simulink model "statespace_verification_sim_model"  (R2016a)
settings: Solver=ode4  StartTime=0.0  StopTime=Tfinal  FixedStep=Ts  RelTol=1e-3
values from neighbouring files (symbols this model uses):
  Cdc = 15e-6    (= 1.5e-05)    [Rectifier.m]    (also in stateSpaceEnes.m; state_space_inverter.m; state_space_inverter_linetolineprinciple.m)
  DCSourceMagn = 300    [Rectifier.m]    (also in state_space_inverter.m; state_space_inverter_linetolineprinciple.m)
  delta = 0    [CapacitorAResponse.m]    (also in Rectifier.m; stateSpaceEnes.m; state_space_inverter.m; state_space_inverter_linetolineprinciple.m)
  fout = 50    [CapacitorAResponse.m]    (also in Rectifier.m; stateSpaceEnes.m; state_space_inverter.m; state_space_inverter_linetolineprinciple.m)
  GridFreq = 50    [Rectifier.m]    (also in state_space_inverter_linetolineprinciple.m)
  LA = 15e-3    (= 0.015)    [CapacitorAResponse.m]    (also in Rectifier.m; stateSpaceEnes.m; state_space_inverter.m; state_space_inverter_linetolineprinciple.m)
  LB = 15e-3    (= 0.015)    [CapacitorAResponse.m]    (also in Rectifier.m; stateSpaceEnes.m; state_space_inverter.m; state_space_inverter_linetolineprinciple.m)
  LC = 15e-3    (= 0.015)    [CapacitorAResponse.m]    (also in Rectifier.m; stateSpaceEnes.m; state_space_inverter.m; state_space_inverter_linetolineprinciple.m)
  Lin = 5e-5    (= 5e-05)    [Rectifier.m]    (also in stateSpaceEnes.m; state_space_inverter.m = 0.001; state_space_inverter_linetolineprinciple.m)
  Lload = 1.1e-3    (= 0.0011)    [fftSwitch.m]
  ma = 0.9    [CapacitorAResponse.m]    (also in Rectifier.m; stateSpaceEnes.m; state_space_inverter.m; state_space_inverter_linetolineprinciple.m)
  RA = 10    [CapacitorAResponse.m]    (also in Rectifier.m; stateSpaceEnes.m; state_space_inverter.m; state_space_inverter_linetolineprinciple.m)
  RB = 10    [CapacitorAResponse.m]    (also in Rectifier.m; stateSpaceEnes.m; state_space_inverter.m; state_space_inverter_linetolineprinciple.m)
  RC = 10    [CapacitorAResponse.m]    (also in Rectifier.m; stateSpaceEnes.m; state_space_inverter.m; state_space_inverter_linetolineprinciple.m)
  Rin = 2    [Rectifier.m]    (also in stateSpaceEnes.m; state_space_inverter.m; state_space_inverter_linetolineprinciple.m)
  Ripth = 0.18    [Rectifier.m]    (also in state_space_inverter.m; state_space_inverter_linetolineprinciple.m)
  Rload = 10    [fftSwitch.m]
  SixthHarmonicFreq = 150    [Rectifier.m]    (also in state_space_inverter.m = 300; state_space_inverter_linetolineprinciple.m = 300)
  SixthHarmonicMagn = DCSourceMagn*(1-0.95262794416)    (= 14.211616752)    [Rectifier.m]    (also in state_space_inverter.m = 0; state_space_inverter_linetolineprinciple.m = 0)
  SixthHarmonicPhase = 0    [Rectifier.m]    (also in state_space_inverter.m; state_space_inverter_linetolineprinciple.m)
  Ts = Tstep    (= 1e-06)    [Rectifier.m]    (also in state_space_inverter.m; state_space_inverter_linetolineprinciple.m)
  Vacrms = 220    [Rectifier.m]    (also in state_space_inverter_linetolineprinciple.m)
libraries: powerlib x39, powerlib_meascontrol x29, simulink x4
settings Model: SimulationMode=accelerator  Creator=ugurm  LastModifiedBy=mesutto
settings DataIOCC: LimitDataPoints=on  SaveFormat=Array
settings DebuggingCC: UnderspecifiedInitializationDetection=Classic  MergeDetectMultiDrivingBlocksExec=none  SolverPrmCheckMsg=warning  StateNameClashWarn=warning
settings HardwareCC: ProdBitPerPointer=32  ProdLargestAtomicFloat=None  ProdIntDivRoundTo=Undefined  ProdEndianess=Unspecified  ProdWordSize=32  ProdHWDeviceType=32-bit Generic
settings ModelReferenceCC: PropagateSignalLabelsOutOfModel=off
settings ConfigComp: CovModelRefEnable=Off

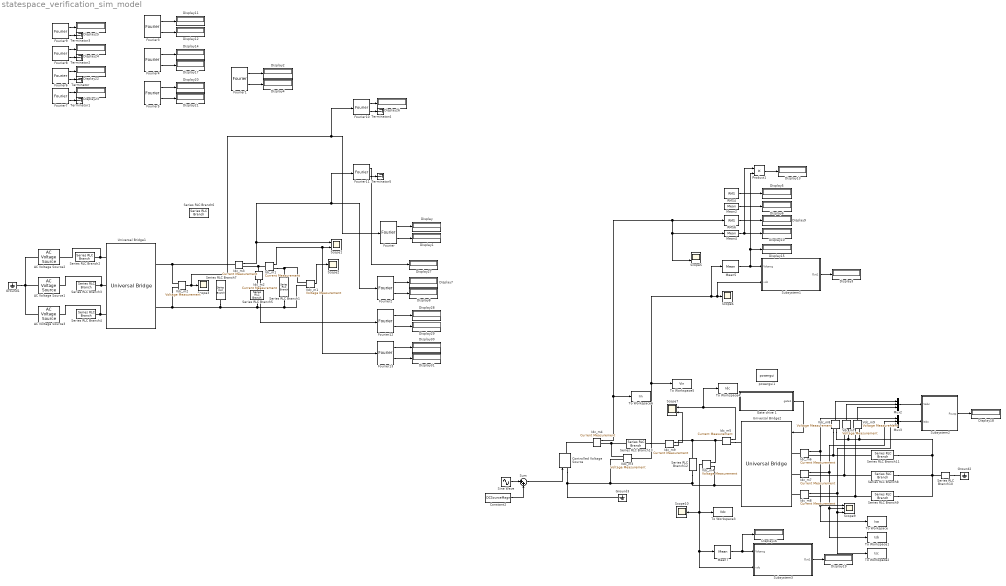
== system statespace_verification_sim_model ==
  AC Voltage Source1 : powerlib/Electrical Sources/AC Voltage Source  Amplitude=Vacrms*sqrt(2)  Phase=-120  Frequency=GridFreq  SampleTime=0  Measurements=None  BusType=swing  Pref=10e3  Qref=0  Qmin=-inf  Qmax=+inf
  AC Voltage Source2 : powerlib/Electrical Sources/AC Voltage Source  Amplitude=Vacrms*sqrt(2)  Phase=0  Frequency=GridFreq  SampleTime=0  Measurements=None  BusType=swing  Pref=10e3  Qref=0  Qmin=-inf  Qmax=+inf
  AC Voltage Source3 : powerlib/Electrical Sources/AC Voltage Source  Amplitude=Vacrms*sqrt(2)  Phase=-240  Frequency=GridFreq  SampleTime=0  Measurements=None  BusType=swing  Pref=10e3  Qref=0  Qmin=-inf  Qmax=+inf
  Constant2 : Constant  Value=DCSourceMagn
  Controlled Voltage Source : powerlib/Electrical Sources/Controlled Voltage Source  Initialize=on  Source_Type=DC  Amplitude=DCSourceMagn  Phase=0  Frequency=0  Measurements=None
  Display{,1..31} (32 alike) : Display
  Fourier{,1..2,12..13} (5 alike) : powerlib_meascontrol/Measurements/Fourier  Freq=GridFreq  n=6  InInit=[0, 0]  Ts=0
  Fourier{6..11} (6 alike) : powerlib_meascontrol/Measurements/Fourier  Freq=GridFreq  n=0  InInit=[0, 0]  Ts=0
  Fourier3 : powerlib_meascontrol/Measurements/Fourier  Freq=GridFreq  n=12  InInit=[0, 0]  Ts=0
  Fourier4 : powerlib_meascontrol/Measurements/Fourier  Freq=GridFreq  n=12  InInit=[0, 0]  Ts=0
  Fourier5 : powerlib_meascontrol/Measurements/Fourier  Freq=GridFreq  n=12  InInit=[0, 0]  Ts=0
  Gate drive 1 : Subsystem
  Ground1 : powerlib/Elements/Ground  LConnTagsString=a
  Ground2 : powerlib/Elements/Ground  LConnTagsString=a
  Ground3 : powerlib/Elements/Ground  LConnTagsString=a
  Idc_m{1..9} (9 alike) : powerlib/Measurements/Current Measurement  PhasorSimulation=off  OutputType=Complex  PSBequivalent=0
  Mean{2,4..5,7} (4 alike) : powerlib_meascontrol/Measurements/Mean  Freq=fout  Vinit=0  Ts=0
  Mux2 : Mux  Inputs=3
  Mux3 : Mux  Inputs=3
  Product1 : Product
  RMS4 : powerlib_meascontrol/Measurements/RMS  TrueRMS=on  Freq=fout  RMSInit=0  Ts=0
  RMS6 : powerlib_meascontrol/Measurements/RMS  TrueRMS=on  Freq=fout  RMSInit=0  Ts=0
  Scope1 : Scope  NumInputPorts=2
  Scope{2..3,6,10} (4 alike) : Scope
  Scope5 : Scope  NumInputPorts=2
  Scope7 : Scope  NumInputPorts=2
  Scope9 : Scope  NumInputPorts=3
  Series RLC Branch1 : powerlib/Elements/Series RLC Branch  LConnTagsString=__new0  RConnTagsString=__new0  BranchType=R  Resistance=50  Inductance=Lin  SetiL0=off  InitialCurrent=0  Capacitance=1e-6  Setx0=off  InitialVoltage=0  Measurements=None
  Series RLC Branch10 : powerlib/Elements/Series RLC Branch  LConnTagsString=__new0  RConnTagsString=__new0  BranchType=R  Resistance=1e12  Inductance=Lload  SetiL0=off  InitialCurrent=0  Capacitance=1e-6  Setx0=off  InitialVoltage=0  Measurements=None
  Series RLC Branch11 : powerlib/Elements/Series RLC Branch  LConnTagsString=__new0  RConnTagsString=__new0  BranchType=RL  Resistance=RA  Inductance=LA  SetiL0=off  InitialCurrent=0  Capacitance=1e-6  Setx0=off  InitialVoltage=0  Measurements=None
  Series RLC Branch12 : powerlib/Elements/Series RLC Branch  LConnTagsString=__new0  RConnTagsString=__new0  BranchType=C  Resistance=Rload  Inductance=Lload  SetiL0=off  InitialCurrent=0  Capacitance=Cdc  Setx0=off  InitialVoltage=0  Measurements=None
  Series RLC Branch13 : powerlib/Elements/Series RLC Branch  LConnTagsString=__new0  RConnTagsString=__new0  BranchType=RL  Resistance=Rin  Inductance=Lin  SetiL0=off  InitialCurrent=0  Capacitance=1e-6  Setx0=off  InitialVoltage=0  Measurements=None
  Series RLC Branch2 : powerlib/Elements/Series RLC Branch  LConnTagsString=__new0  RConnTagsString=__new0  BranchType=RL  Resistance=1e-3  Inductance=1e-6  SetiL0=off  InitialCurrent=0  Capacitance=1e-6  Setx0=off  InitialVoltage=0  Measurements=None
  Series RLC Branch3 : powerlib/Elements/Series RLC Branch  LConnTagsString=__new0  RConnTagsString=__new0  BranchType=RL  Resistance=1e-3  Inductance=1e-6  SetiL0=off  InitialCurrent=0  Capacitance=1e-6  Setx0=off  InitialVoltage=0  Measurements=None
  Series RLC Branch4 : powerlib/Elements/Series RLC Branch  LConnTagsString=__new0  RConnTagsString=__new0  BranchType=RL  Resistance=1e-3  Inductance=1e-6  SetiL0=off  InitialCurrent=0  Capacitance=1e-6  Setx0=off  InitialVoltage=0  Measurements=None
  Series RLC Branch5 : powerlib/Elements/Series RLC Branch  LConnTagsString=__new0  RConnTagsString=__new0  BranchType=C  Resistance=Rload  Inductance=Lload  SetiL0=off  InitialCurrent=0  Capacitance=15e-3  Setx0=on  InitialVoltage=540  Measurements=None
  Series RLC Branch6 : powerlib/Elements/Series RLC Branch  LConnTagsString=__new0  RConnTagsString=__new0  BranchType=R  Resistance=0.5  Inductance=Lin  SetiL0=off  InitialCurrent=0  Capacitance=1e-6  Setx0=off  InitialVoltage=0  Measurements=None
  Series RLC Branch7 : powerlib/Elements/Series RLC Branch  LConnTagsString=__new0  RConnTagsString=__new0  BranchType=R  Resistance=1  Inductance=Lin  SetiL0=off  InitialCurrent=0  Capacitance=1e-6  Setx0=off  InitialVoltage=0  Measurements=None
  Series RLC Branch8 : powerlib/Elements/Series RLC Branch  LConnTagsString=__new0  RConnTagsString=__new0  BranchType=RL  Resistance=RB  Inductance=LB  SetiL0=off  InitialCurrent=0  Capacitance=1e-6  Setx0=off  InitialVoltage=0  Measurements=None
  Series RLC Branch9 : powerlib/Elements/Series RLC Branch  LConnTagsString=__new0  RConnTagsString=__new0  BranchType=RL  Resistance=RC  Inductance=LC  SetiL0=off  InitialCurrent=0  Capacitance=1e-6  Setx0=off  InitialVoltage=0  Measurements=None
  Sine Wave : Sin  Amplitude=SixthHarmonicMagn  Frequency=2*pi*SixthHarmonicFreq  Phase=SixthHarmonicPhase  SampleTime=0
  Subsystem1 : Subsystem
  Subsystem2 : Subsystem
  Subsystem3 : Subsystem
  Sum : Sum  Inputs=|++
  Terminator{,1..5} (6 alike) : Terminator
  To Workspace : ToWorkspace  VariableName=Isa  SampleTime=-1
  To Workspace1 : ToWorkspace  VariableName=Isb  SampleTime=-1
  To Workspace2 : ToWorkspace  VariableName=Isc  SampleTime=-1
  To Workspace3 : ToWorkspace  VariableName=Vdc  SampleTime=-1
  To Workspace4 : ToWorkspace  VariableName=Idc  SampleTime=-1
  To Workspace5 : ToWorkspace  VariableName=Vin  SampleTime=-1
  To Workspace6 : ToWorkspace  VariableName=Iin  SampleTime=-1
  Universal Bridge1 : powerlib/Power Electronics/Universal Bridge  Arms=3  SnubberResistance=1e5  SnubberCapacitance=inf  Device=Diodes  Ron=1e-6  Lon=0  ForwardVoltages="[  0  0  ]"  ForwardVoltage=0  GTOparameters=[ 10e-6 , 20e-6 ]  IGBTparameters=[0,0]  Measurements=None  Measurements_2=None  converterType=Rectifier
  Universal Bridge2 : powerlib/Power Electronics/Universal Bridge  Arms=3  SnubberResistance=1e5  SnubberCapacitance=inf  Device=IGBT / Diodes  Ron=1e-6  Lon=0  ForwardVoltages="[  0  0  ]"  ForwardVoltage=0  GTOparameters=[ 10e-6 , 20e-6 ]  IGBTparameters=[0,0]  Measurements=None  Measurements_2=None  converterType=Rectifier
  Vdc_m{1..4,7..9} (7 alike) : powerlib/Measurements/Voltage Measurement  PhasorSimulation=off  OutputType=Complex  PSBequivalent=0
  powergui1 : powerlib/powergui  Priority=1  SimulationMode=Discrete  SolverType=Tustin  SampleTime=Ts  frequency=60  SPID=off  DisableSnubberDevices=off  DisableRonSwitches=off  DisableVfSwitches=off  SwTol=0  DisplayEquations=off  Interpol=off  ExternalGateDelay=off  methode=off  Ts=0  FunctionMessages=off  echomessages=off  HookPort=off  EnableUseOfTLC=off  x0status=blocks  frequencyindice=0  Pbase=100e6  ErrMax=1e-4  Iterations=50  UnitsV=kV  UnitsW=MW  buscounter=0  RestoreLinks=warning  ResistiveCurrentMeasurement=off  Frange=[0:2:500]  Ylog=off  Xlog=on  ShowGrid=off  save=off  variable=ZData  structure=idcrec  ZoomFFT=off  StartTime=0.02  cycles=4  DisplayStyle=6  fundamental=50  FreqAxis=off  MaxFrequency=2000  frequencyindicesteady=1  RmsSteady=1  display=off
  wires:
  Idc_m4/1 -> To Workspace6/1, Scope5/2, Mean4/1, RMS6/1
  Vdc_m3/1 -> Mean5/1, Subsystem1/2(vdc), Scope6/1, To Workspace5/1
  Mean5/1 -> Display15/1, Product1/2, Subsystem1/1(Vdcavg)
  Subsystem1/1(Out1) -> Display3/1
  RMS4/1 -> Display5/1
  Mean2/1 -> Display6/1
  Mean4/1 -> Product1/1, Display10/1
  RMS6/1 -> Display9/1
  Product1/1 -> Display13/1
  Gate drive 1/1(gate1) -> Universal Bridge2/1
  Idc_m6/1 -> Mux3/1, To Workspace/1, Scope9/1
  Idc_m7/1 -> Mux3/2, To Workspace1/1, Scope9/2
  Idc_m8/1 -> Scope9/3, To Workspace2/1, Mux3/3
  Vdc_m8/1 -> Mux2/1
  Vdc_m7/1 -> Mux2/2
  Vdc_m9/1 -> Mux2/3
  Mux2/1 -> Subsystem2/1(Vabc)
  Mux3/1 -> Subsystem2/2(Iabc)
  Subsystem2/1(Poutp) -> Display18/1
  Idc_m5/1 -> To Workspace4/1, Scope7/1
  Idc_m9/1 -> Scope7/2
  Vdc_m4/1 -> To Workspace3/1, Mean7/1, Subsystem3/2(vdc), Scope10/1
  Mean7/1 -> Display16/1, Subsystem3/1(Vdcavg)
  Subsystem3/1(Out1) -> Display19/1
  Sine Wave/1 -> Sum/1
  Constant2/1 -> Sum/2
  Sum/1 -> Controlled Voltage Source/1
  Idc_m3/1 -> Fourier11/1, Fourier2/1, Scope1/1
  Fourier/1 -> Display/1
  Fourier/2 -> Display1/1
  Fourier1/1 -> Display2/1
  Fourier1/2 -> Display4/1
  Fourier2/1 -> Display7/1
  Fourier2/2 -> Display8/1
  Fourier3/1 -> Display11/1
  Fourier3/2 -> Display12/1
  Fourier4/1 -> Display14/1
  Fourier4/2 -> Display17/1
  Fourier5/1 -> Display20/1
  Fourier5/2 -> Display21/1
  Fourier6/2 -> Terminator/1
  Fourier6/1 -> Display22/1
  Idc_m1/1 -> Fourier13/1, Scope1/2
  Fourier7/2 -> Terminator1/1
  Fourier7/1 -> Display23/1
  Vdc_m2/1 -> Fourier10/1, Fourier/1, Scope3/1
  Fourier8/2 -> Terminator2/1
  Fourier8/1 -> Display24/1
  Fourier9/2 -> Terminator3/1
  Fourier9/1 -> Display25/1
  Vdc_m1/1 -> Scope2/1
  Fourier10/2 -> Terminator4/1
  Fourier10/1 -> Display26/1
  Fourier11/2 -> Terminator5/1
  Fourier11/1 -> Display27/1
  Fourier12/1 -> Display28/1
  Fourier12/2 -> Display29/1
  Idc_m2/1 -> Fourier12/1
  Fourier13/1 -> Display30/1
  Fourier13/2 -> Display31/1
  connections:
  Series RLC Branch3/RConn1 -- AC Voltage Source1/RConn1 -- Universal Bridge1/LConn2
  Universal Bridge1/LConn1 -- AC Voltage Source2/RConn1 -- Series RLC Branch2/RConn1
  Ground1/LConn1 -- AC Voltage Source3/LConn1 -- AC Voltage Source2/LConn1 -- AC Voltage Source1/LConn1
  Idc_m1/LConn1 -- Idc_m2/LConn1 -- Idc_m3/RConn1
  Vdc_m2/LConn1 -- Idc_m3/LConn1 -- Universal Bridge1/RConn1
  Idc_m5/LConn1 -- Idc_m9/RConn1 -- Series RLC Branch12/LConn1 -- Vdc_m4/LConn1
  Idc_m6/RConn1 -- Vdc_m8/LConn1 -- Series RLC Branch11/LConn1
  Series RLC Branch9/RConn1 -- Series RLC Branch10/LConn1 -- Vdc_m8/LConn2 -- Vdc_m7/LConn2 -- Vdc_m9/LConn2 -- Series RLC Branch11/RConn1 -- Series RLC Branch8/RConn1
  Idc_m8/RConn1 -- Series RLC Branch9/LConn1 -- Vdc_m9/LConn1
  Idc_m7/RConn1 -- Series RLC Branch8/LConn1 -- Vdc_m7/LConn1
  Idc_m6/LConn1 -- Universal Bridge2/LConn1
  Idc_m5/RConn1 -- Universal Bridge2/RConn1
  Series RLC Branch10/RConn1 -- Ground2/LConn1
  Idc_m8/LConn1 -- Universal Bridge2/LConn3
  Idc_m7/LConn1 -- Universal Bridge2/LConn2
  Series RLC Branch13/LConn1 -- Vdc_m3/LConn1 -- Idc_m4/RConn1
  Series RLC Branch13/RConn1 -- Idc_m9/LConn1
  Series RLC Branch5/RConn1 -- Series RLC Branch1/RConn1 -- Vdc_m1/LConn2 -- Series RLC Branch7/RConn1 -- Vdc_m2/LConn2 -- Universal Bridge1/RConn2
  Controlled Voltage Source/RConn1 -- Idc_m4/LConn1
  Universal Bridge2/RConn2 -- Ground3/LConn1 -- Controlled Voltage Source/LConn1 -- Vdc_m3/LConn2 -- Series RLC Branch12/RConn1 -- Vdc_m4/LConn2
  Vdc_m1/LConn1 -- Idc_m1/RConn1 -- Series RLC Branch1/LConn1
  Series RLC Branch4/RConn1 -- AC Voltage Source3/RConn1 -- Universal Bridge1/LConn3
  Idc_m2/RConn1 -- Series RLC Branch5/LConn1

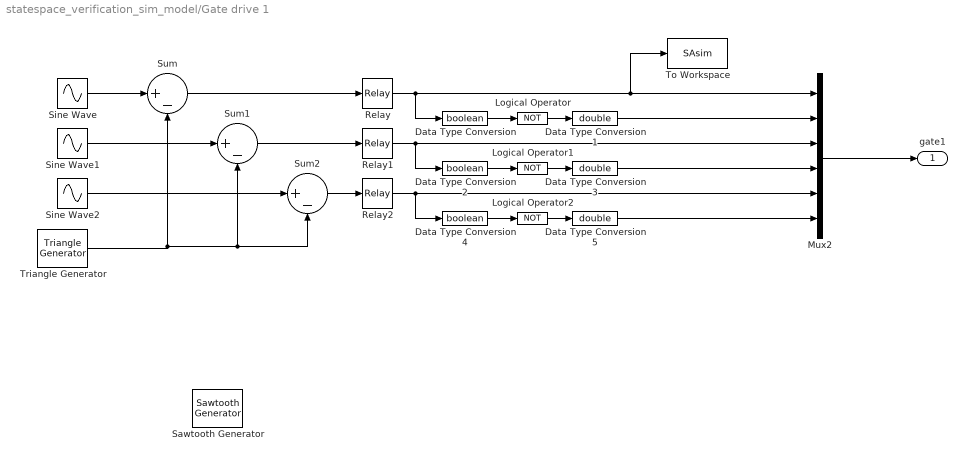
== system statespace_verification_sim_model/Gate drive 1 ==
  Data Type Conversion : DataTypeConversion  OutDataTypeStr=boolean
  Data Type Conversion1 : DataTypeConversion  OutDataTypeStr=double
  Data Type Conversion2 : DataTypeConversion  OutDataTypeStr=boolean
  Data Type Conversion3 : DataTypeConversion  OutDataTypeStr=double
  Data Type Conversion4 : DataTypeConversion  OutDataTypeStr=boolean
  Data Type Conversion5 : DataTypeConversion  OutDataTypeStr=double
  Logical Operator : Logic  Operator=NOT  AllPortsSameDT=off  OutDataTypeStr=boolean
  Logical Operator1 : Logic  Operator=NOT  AllPortsSameDT=off  OutDataTypeStr=boolean
  Logical Operator2 : Logic  Operator=NOT  AllPortsSameDT=off  OutDataTypeStr=boolean
  Mux2 : Mux  Inputs=6
  Relay : Relay
  Relay1 : Relay
  Relay2 : Relay
  Sawtooth Generator : powerlib_meascontrol/Pulse & Signal Generators/Sawtooth Generator  Freq=fsw  Phase=0  Ts=0
  Sine Wave : Sin  Amplitude=ma  Frequency=2*pi*fout  Phase=delta  SampleTime=0
  Sine Wave1 : Sin  Amplitude=ma  Frequency=2*pi*fout  Phase=-2*pi/3+delta  SampleTime=0
  Sine Wave2 : Sin  Amplitude=ma  Frequency=2*pi*fout  Phase=2*pi/3+delta  SampleTime=0
  Sum : Sum  Inputs=|+-
  Sum1 : Sum  Inputs=|+-
  Sum2 : Sum  Inputs=|+-
  To Workspace : ToWorkspace  VariableName=SAsim  SampleTime=-1
  Triangle Generator : powerlib_meascontrol/Pulse & Signal Generators/Triangle Generator  Freq=fsw  Phase=0  Ts=Ts
  gate1 : Outport
  wires:
  Sine Wave/1 -> Sum/1
  Triangle Generator/1 -> Sum1/2, Sum2/2, Sum/2
  Sine Wave1/1 -> Sum1/1
  Sine Wave2/1 -> Sum2/1
  Sum/1 -> Relay/1
  Sum1/1 -> Relay1/1
  Sum2/1 -> Relay2/1
  Data Type Conversion/1 -> Logical Operator/1
  Relay/1 -> Data Type Conversion/1, To Workspace/1, Mux2/1
  Logical Operator/1 -> Data Type Conversion1/1
  Data Type Conversion1/1 -> Mux2/2
  Data Type Conversion2/1 -> Logical Operator1/1
  Relay1/1 -> Data Type Conversion2/1, Mux2/3
  Logical Operator1/1 -> Data Type Conversion3/1
  Data Type Conversion3/1 -> Mux2/4
  Data Type Conversion4/1 -> Logical Operator2/1
  Relay2/1 -> Data Type Conversion4/1, Mux2/5
  Logical Operator2/1 -> Data Type Conversion5/1
  Data Type Conversion5/1 -> Mux2/6
  Mux2/1 -> gate1/1

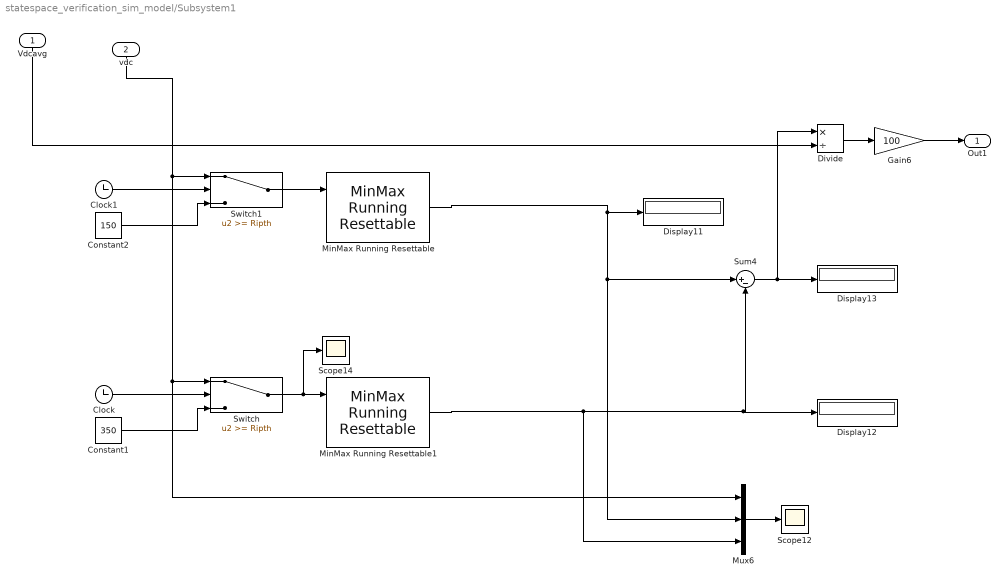
== system statespace_verification_sim_model/Subsystem1 ==
  Vdcavg : Inport
  vdc : Inport  Port=2
  Clock : Clock
  Clock1 : Clock
  Constant1 : Constant  Value=350  SampleTime=Ts
  Constant2 : Constant  Value=150  SampleTime=Ts
  Display11 : Display
  Display12 : Display
  Display13 : Display
  Divide : Product  Inputs=*/
  Gain6 : Gain  Gain=100
  MinMax Running Resettable : simulink/Math Operations/MinMax Running Resettable  Function=max  vinit=0.0
  MinMax Running Resettable1 : simulink/Math Operations/MinMax Running Resettable  Function=min  vinit=700
  Mux6 : Mux  Inputs=3
  Scope12 : Scope
  Scope14 : Scope
  Sum4 : Sum  Inputs=|+-
  Switch : Switch  Threshold=Ripth
  Switch1 : Switch  Threshold=Ripth
  Out1 : Outport
  wires:
  MinMax Running Resettable/1 -> Display11/1, Mux6/2, Sum4/1
  Clock/1 -> Switch/2
  Gain6/1 -> Out1/1
  Constant1/1 -> Switch/3
  MinMax Running Resettable1/1 -> Mux6/3, Display12/1, Sum4/2
  Switch/1 -> Scope14/1, MinMax Running Resettable1/1
  Sum4/1 -> Divide/1, Display13/1
  Divide/1 -> Gain6/1
  Mux6/1 -> Scope12/1
  Vdcavg/1 -> Divide/2
  vdc/1 -> Switch1/1, Mux6/1, Switch/1
  Switch1/1 -> MinMax Running Resettable/1
  Clock1/1 -> Switch1/2
  Constant2/1 -> Switch1/3

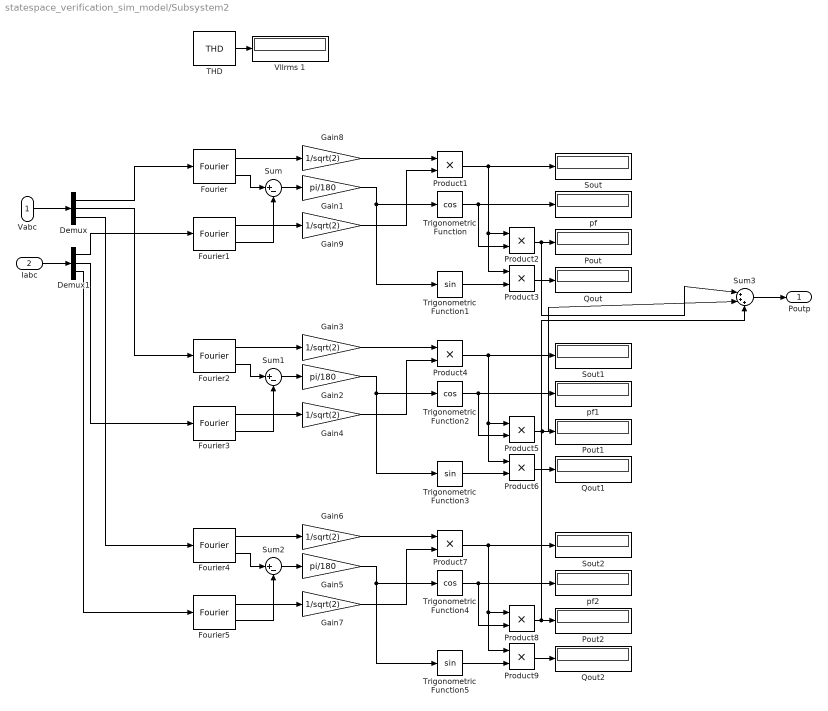
== system statespace_verification_sim_model/Subsystem2 ==
  Vabc : Inport
  Iabc : Inport  Port=2
  Demux : Demux  Outputs=3
  Demux1 : Demux  Outputs=3
  Fourier{,1..5} (6 alike) : powerlib_meascontrol/Measurements/Fourier  Freq=fout  n=1  InInit=[0, 0]  Ts=Ts
  Gain1 : Gain  Gain=pi/180
  Gain2 : Gain  Gain=pi/180
  Gain{3..4,6..9} (6 alike) : Gain  Gain=1/sqrt(2)
  Gain5 : Gain  Gain=pi/180
  Pout : Display
  Pout1 : Display
  Pout2 : Display
  Product{1..9} (9 alike) : Product
  Qout : Display
  Qout1 : Display
  Qout2 : Display
  Sout : Display
      settings: Format=short_e
  Sout1 : Display
      settings: Format=short_e
  Sout2 : Display
      settings: Format=short_e
  Sum : Sum  Inputs=|+-
  Sum1 : Sum  Inputs=|+-
  Sum2 : Sum  Inputs=|+-
  Sum3 : Sum  Inputs=|+++
  THD : powerlib_meascontrol/Measurements/THD  Freq=fout  Ts=0
  Trigonometric Function : Trigonometry  Operator=cos
  Trigonometric Function1 : Trigonometry
  Trigonometric Function2 : Trigonometry  Operator=cos
  Trigonometric Function3 : Trigonometry
  Trigonometric Function4 : Trigonometry  Operator=cos
  Trigonometric Function5 : Trigonometry
  Vllrms 1 : Display
  pf : Display
  pf1 : Display
  pf2 : Display
  Poutp : Outport
  wires:
  Gain8/1 -> Product1/1
  Gain9/1 -> Product1/2
  Fourier1/1 -> Gain9/1
  Fourier/1 -> Gain8/1
  Product1/1 -> Product3/1, Product2/1, Sout/1
  Sum/1 -> Gain1/1
  Trigonometric Function/1 -> Product2/2, pf/1
  Gain1/1 -> Trigonometric Function1/1, Trigonometric Function/1
  Product2/1 -> Sum3/1, Pout/1
  THD/1 -> Vllrms 1/1
  Vabc/1 -> Demux/1
  Iabc/1 -> Demux1/1
  Fourier/2 -> Sum/1
  Fourier1/2 -> Sum/2
  Trigonometric Function1/1 -> Product3/2
  Product3/1 -> Qout/1
  Gain3/1 -> Product4/1
  Gain4/1 -> Product4/2
  Fourier3/1 -> Gain4/1
  Fourier2/1 -> Gain3/1
  Product4/1 -> Product6/1, Product5/1, Sout1/1
  Sum1/1 -> Gain2/1
  Trigonometric Function2/1 -> Product5/2, pf1/1
  Gain2/1 -> Trigonometric Function3/1, Trigonometric Function2/1
  Product5/1 -> Sum3/2, Pout1/1
  Fourier2/2 -> Sum1/1
  Fourier3/2 -> Sum1/2
  Trigonometric Function3/1 -> Product6/2
  Product6/1 -> Qout1/1
  Gain6/1 -> Product7/1
  Gain7/1 -> Product7/2
  Fourier5/1 -> Gain7/1
  Fourier4/1 -> Gain6/1
  Product7/1 -> Product9/1, Product8/1, Sout2/1
  Sum2/1 -> Gain5/1
  Trigonometric Function4/1 -> Product8/2, pf2/1
  Gain5/1 -> Trigonometric Function5/1, Trigonometric Function4/1
  Fourier4/2 -> Sum2/1
  Fourier5/2 -> Sum2/2
  Trigonometric Function5/1 -> Product9/2
  Product9/1 -> Qout2/1
  Product8/1 -> Sum3/3, Pout2/1
  Sum3/1 -> Poutp/1
  Demux/1 -> Fourier/1
  Demux/2 -> Fourier2/1
  Demux/3 -> Fourier4/1
  Demux1/1 -> Fourier1/1
  Demux1/2 -> Fourier3/1
  Demux1/3 -> Fourier5/1

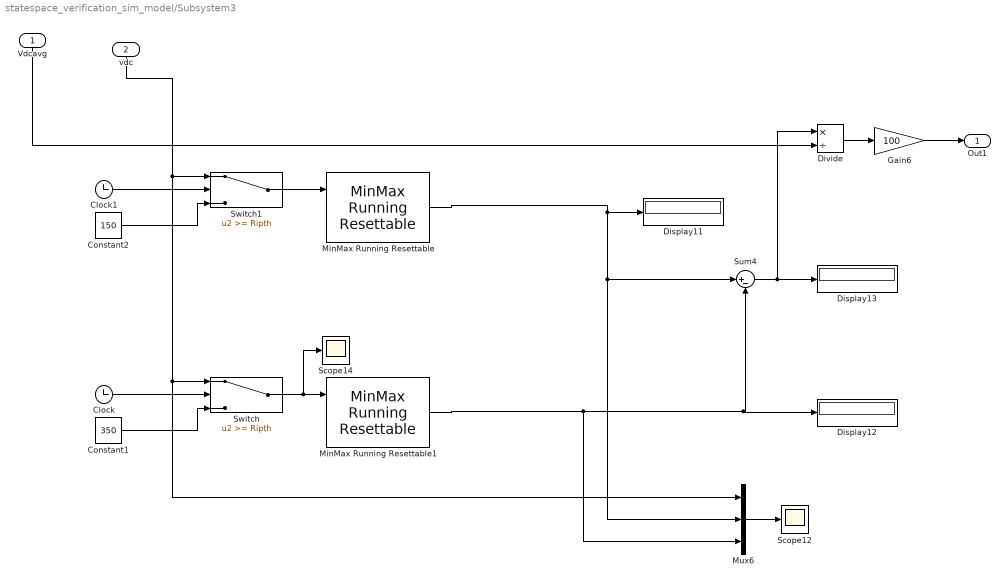
== system statespace_verification_sim_model/Subsystem3 ==
  Vdcavg : Inport
  vdc : Inport  Port=2
  Clock : Clock
  Clock1 : Clock
  Constant1 : Constant  Value=350  SampleTime=Ts
  Constant2 : Constant  Value=150  SampleTime=Ts
  Display11 : Display
  Display12 : Display
  Display13 : Display
  Divide : Product  Inputs=*/
  Gain6 : Gain  Gain=100
  MinMax Running Resettable : simulink/Math Operations/MinMax Running Resettable  Function=max  vinit=0.0
  MinMax Running Resettable1 : simulink/Math Operations/MinMax Running Resettable  Function=min  vinit=700
  Mux6 : Mux  Inputs=3
  Scope12 : Scope
  Scope14 : Scope
  Sum4 : Sum  Inputs=|+-
  Switch : Switch  Threshold=Ripth
  Switch1 : Switch  Threshold=Ripth
  Out1 : Outport
  wires:
  MinMax Running Resettable/1 -> Display11/1, Mux6/2, Sum4/1
  Clock/1 -> Switch/2
  Gain6/1 -> Out1/1
  Constant1/1 -> Switch/3
  MinMax Running Resettable1/1 -> Mux6/3, Display12/1, Sum4/2
  Switch/1 -> Scope14/1, MinMax Running Resettable1/1
  Sum4/1 -> Divide/1, Display13/1
  Divide/1 -> Gain6/1
  Mux6/1 -> Scope12/1
  Vdcavg/1 -> Divide/2
  vdc/1 -> Switch1/1, Mux6/1, Switch/1
  Switch1/1 -> MinMax Running Resettable/1
  Clock1/1 -> Switch1/2
  Constant2/1 -> Switch1/3
